simulink model "Battery_model"  (R2021b)
settings: Solver=FixedStepAuto  StartTime=0.0  StopTime=mdl_input.t(end)  FixedStep=1  RelTol=1e-3
values from neighbouring files (symbols this model uses):
  params =     [cell_param.mat]
undefined symbols (not defined in the file or in its folder): mdl_input
libraries: fl_lib x78, nesl_utility x77, simulink x14, ee_lib x14
(part 2 of 2)

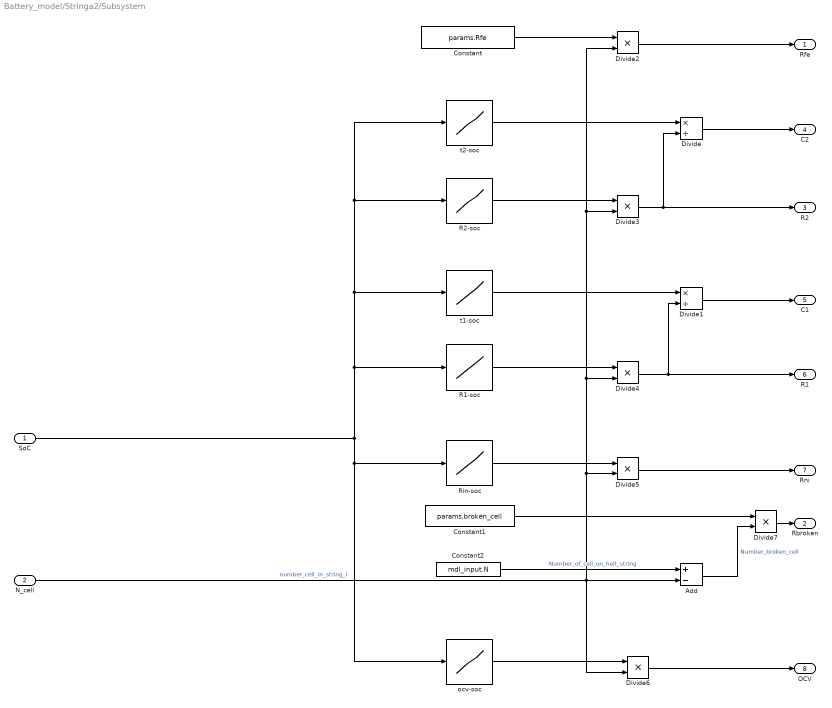
== system Battery_model/Stringa2/Subsystem ==
  SoC : Inport
  N_cell : Inport  Port=2
  Add : Sum  Inputs=+-
  Constant : Constant  Value=params.Rfe
  Constant1 : Constant  Value=params.broken_cell
  Constant2 : Constant  Value=mdl_input.N
  Divide : Product  Inputs=*/
  Divide1 : Product  Inputs=*/
  Divide{2..7} (6 alike) : Product  Inputs=**
  R1-soc : Lookup_n-D  NumberOfTableDimensions=1  BreakpointsForDimension1=params.SoC  Table=params.R1  InternalRulePriority=Speed  RndMeth=Simplest  InputSameDT=on
  R2-soc : Lookup_n-D  NumberOfTableDimensions=1  BreakpointsForDimension1=params.SoC  Table=params.R2  InternalRulePriority=Speed  RndMeth=Simplest  InputSameDT=on
  Rin-soc : Lookup_n-D  NumberOfTableDimensions=1  BreakpointsForDimension1=params.SoC  Table=params.Rni  InternalRulePriority=Speed  RndMeth=Simplest  InputSameDT=on
  ocv-soc : Lookup_n-D  NumberOfTableDimensions=1  BreakpointsForDimension1=params.SoC  Table=params.OCV  ExtrapMethod=Clip  UseLastTableValue=on  InternalRulePriority=Speed  RndMeth=Simplest  InputSameDT=on
  t1-soc : Lookup_n-D  NumberOfTableDimensions=1  BreakpointsForDimension1=params.SoC  Table=params.t1  InternalRulePriority=Speed  RndMeth=Simplest  InputSameDT=on
  t2-soc : Lookup_n-D  NumberOfTableDimensions=1  BreakpointsForDimension1=params.SoC  Table=params.t2  InternalRulePriority=Speed  RndMeth=Simplest  InputSameDT=on
  Rfe : Outport
  Rbroken : Outport  Port=2
  R2 : Outport  Port=3
  C2 : Outport  Port=4
  C1 : Outport  Port=5
  R1 : Outport  Port=6
  Rni : Outport  Port=7
  OCV : Outport  Port=8
  wires:
  SoC/1 -> ocv-soc/1, Rin-soc/1, t1-soc/1, R2-soc/1, t2-soc/1, R1-soc/1
  t1-soc/1 -> Divide1/1
  Divide1/1 -> C1/1
  t2-soc/1 -> Divide/1
  Divide/1 -> C2/1
  Constant/1 -> Divide2/1
  Divide2/1 -> Rfe/1
  R2-soc/1 -> Divide3/1
  Divide3/1 -> Divide/2, R2/1
  Divide4/1 -> Divide1/2, R1/1
  R1-soc/1 -> Divide4/1
  ocv-soc/1 -> Divide6/1
  Divide6/1 -> OCV/1
  Rin-soc/1 -> Divide5/1
  N_cell/1 -> Divide6/2, Add/2, Divide5/2, Divide4/2, Divide3/2, Divide2/2  "number_cell_in_string_i"
  Constant2/1 -> Add/1  "Number_of_cell_on_helt_string"
  Constant1/1 -> Divide7/1
  Add/1 -> Divide7/2  "Number_broken_cell"
  Divide7/1 -> Rbroken/1
  Divide5/1 -> Rni/1

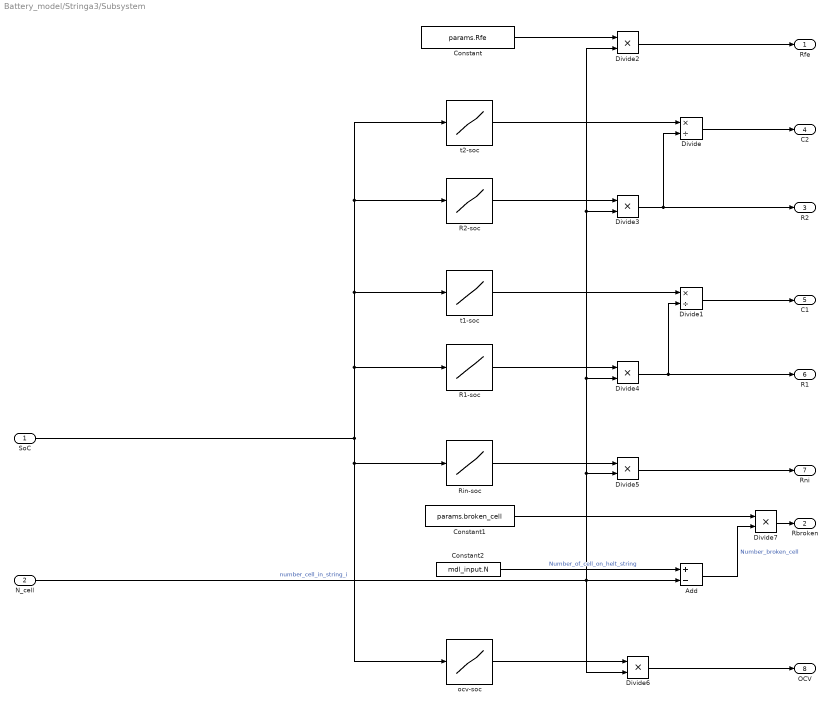
== system Battery_model/Stringa3/Subsystem ==
  SoC : Inport
  N_cell : Inport  Port=2
  Add : Sum  Inputs=+-
  Constant : Constant  Value=params.Rfe
  Constant1 : Constant  Value=params.broken_cell
  Constant2 : Constant  Value=mdl_input.N
  Divide : Product  Inputs=*/
  Divide1 : Product  Inputs=*/
  Divide{2..7} (6 alike) : Product  Inputs=**
  R1-soc : Lookup_n-D  NumberOfTableDimensions=1  BreakpointsForDimension1=params.SoC  Table=params.R1  InternalRulePriority=Speed  RndMeth=Simplest  InputSameDT=on
  R2-soc : Lookup_n-D  NumberOfTableDimensions=1  BreakpointsForDimension1=params.SoC  Table=params.R2  InternalRulePriority=Speed  RndMeth=Simplest  InputSameDT=on
  Rin-soc : Lookup_n-D  NumberOfTableDimensions=1  BreakpointsForDimension1=params.SoC  Table=params.Rni  InternalRulePriority=Speed  RndMeth=Simplest  InputSameDT=on
  ocv-soc : Lookup_n-D  NumberOfTableDimensions=1  BreakpointsForDimension1=params.SoC  Table=params.OCV  ExtrapMethod=Clip  UseLastTableValue=on  InternalRulePriority=Speed  RndMeth=Simplest  InputSameDT=on
  t1-soc : Lookup_n-D  NumberOfTableDimensions=1  BreakpointsForDimension1=params.SoC  Table=params.t1  InternalRulePriority=Speed  RndMeth=Simplest  InputSameDT=on
  t2-soc : Lookup_n-D  NumberOfTableDimensions=1  BreakpointsForDimension1=params.SoC  Table=params.t2  InternalRulePriority=Speed  RndMeth=Simplest  InputSameDT=on
  Rfe : Outport
  Rbroken : Outport  Port=2
  R2 : Outport  Port=3
  C2 : Outport  Port=4
  C1 : Outport  Port=5
  R1 : Outport  Port=6
  Rni : Outport  Port=7
  OCV : Outport  Port=8
  wires:
  SoC/1 -> ocv-soc/1, Rin-soc/1, t1-soc/1, R2-soc/1, t2-soc/1, R1-soc/1
  t1-soc/1 -> Divide1/1
  Divide1/1 -> C1/1
  t2-soc/1 -> Divide/1
  Divide/1 -> C2/1
  Constant/1 -> Divide2/1
  Divide2/1 -> Rfe/1
  R2-soc/1 -> Divide3/1
  Divide3/1 -> Divide/2, R2/1
  Divide4/1 -> Divide1/2, R1/1
  R1-soc/1 -> Divide4/1
  ocv-soc/1 -> Divide6/1
  Divide6/1 -> OCV/1
  Rin-soc/1 -> Divide5/1
  N_cell/1 -> Divide6/2, Add/2, Divide5/2, Divide4/2, Divide3/2, Divide2/2  "number_cell_in_string_i"
  Constant2/1 -> Add/1  "Number_of_cell_on_helt_string"
  Constant1/1 -> Divide7/1
  Add/1 -> Divide7/2  "Number_broken_cell"
  Divide7/1 -> Rbroken/1
  Divide5/1 -> Rni/1

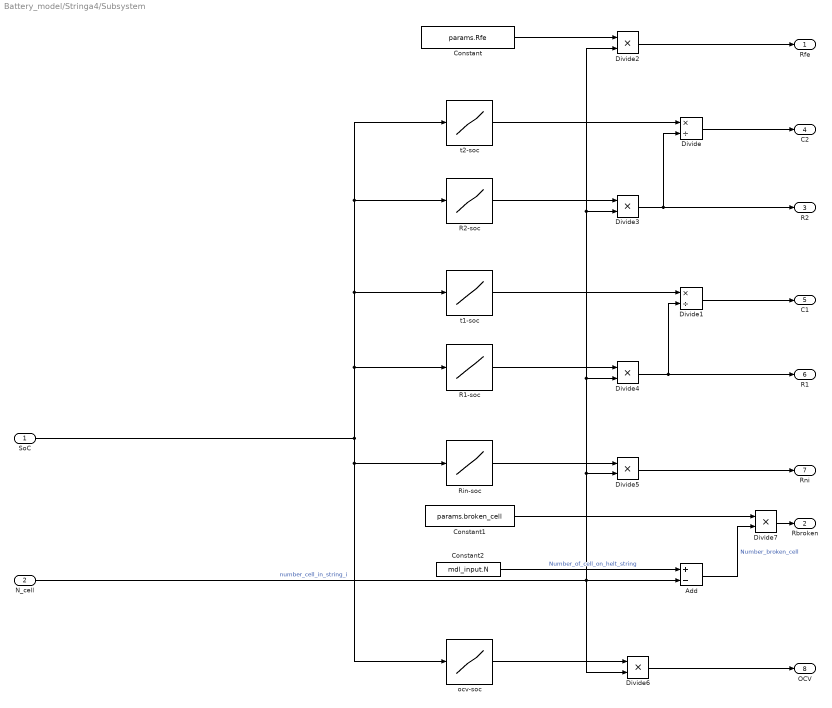
== system Battery_model/Stringa4/Subsystem ==
  SoC : Inport
  N_cell : Inport  Port=2
  Add : Sum  Inputs=+-
  Constant : Constant  Value=params.Rfe
  Constant1 : Constant  Value=params.broken_cell
  Constant2 : Constant  Value=mdl_input.N
  Divide : Product  Inputs=*/
  Divide1 : Product  Inputs=*/
  Divide{2..7} (6 alike) : Product  Inputs=**
  R1-soc : Lookup_n-D  NumberOfTableDimensions=1  BreakpointsForDimension1=params.SoC  Table=params.R1  InternalRulePriority=Speed  RndMeth=Simplest  InputSameDT=on
  R2-soc : Lookup_n-D  NumberOfTableDimensions=1  BreakpointsForDimension1=params.SoC  Table=params.R2  InternalRulePriority=Speed  RndMeth=Simplest  InputSameDT=on
  Rin-soc : Lookup_n-D  NumberOfTableDimensions=1  BreakpointsForDimension1=params.SoC  Table=params.Rni  InternalRulePriority=Speed  RndMeth=Simplest  InputSameDT=on
  ocv-soc : Lookup_n-D  NumberOfTableDimensions=1  BreakpointsForDimension1=params.SoC  Table=params.OCV  ExtrapMethod=Clip  UseLastTableValue=on  InternalRulePriority=Speed  RndMeth=Simplest  InputSameDT=on
  t1-soc : Lookup_n-D  NumberOfTableDimensions=1  BreakpointsForDimension1=params.SoC  Table=params.t1  InternalRulePriority=Speed  RndMeth=Simplest  InputSameDT=on
  t2-soc : Lookup_n-D  NumberOfTableDimensions=1  BreakpointsForDimension1=params.SoC  Table=params.t2  InternalRulePriority=Speed  RndMeth=Simplest  InputSameDT=on
  Rfe : Outport
  Rbroken : Outport  Port=2
  R2 : Outport  Port=3
  C2 : Outport  Port=4
  C1 : Outport  Port=5
  R1 : Outport  Port=6
  Rni : Outport  Port=7
  OCV : Outport  Port=8
  wires:
  SoC/1 -> ocv-soc/1, Rin-soc/1, t1-soc/1, R2-soc/1, t2-soc/1, R1-soc/1
  t1-soc/1 -> Divide1/1
  Divide1/1 -> C1/1
  t2-soc/1 -> Divide/1
  Divide/1 -> C2/1
  Constant/1 -> Divide2/1
  Divide2/1 -> Rfe/1
  R2-soc/1 -> Divide3/1
  Divide3/1 -> Divide/2, R2/1
  Divide4/1 -> Divide1/2, R1/1
  R1-soc/1 -> Divide4/1
  ocv-soc/1 -> Divide6/1
  Divide6/1 -> OCV/1
  Rin-soc/1 -> Divide5/1
  N_cell/1 -> Divide6/2, Add/2, Divide5/2, Divide4/2, Divide3/2, Divide2/2  "number_cell_in_string_i"
  Constant2/1 -> Add/1  "Number_of_cell_on_helt_string"
  Constant1/1 -> Divide7/1
  Add/1 -> Divide7/2  "Number_broken_cell"
  Divide7/1 -> Rbroken/1
  Divide5/1 -> Rni/1

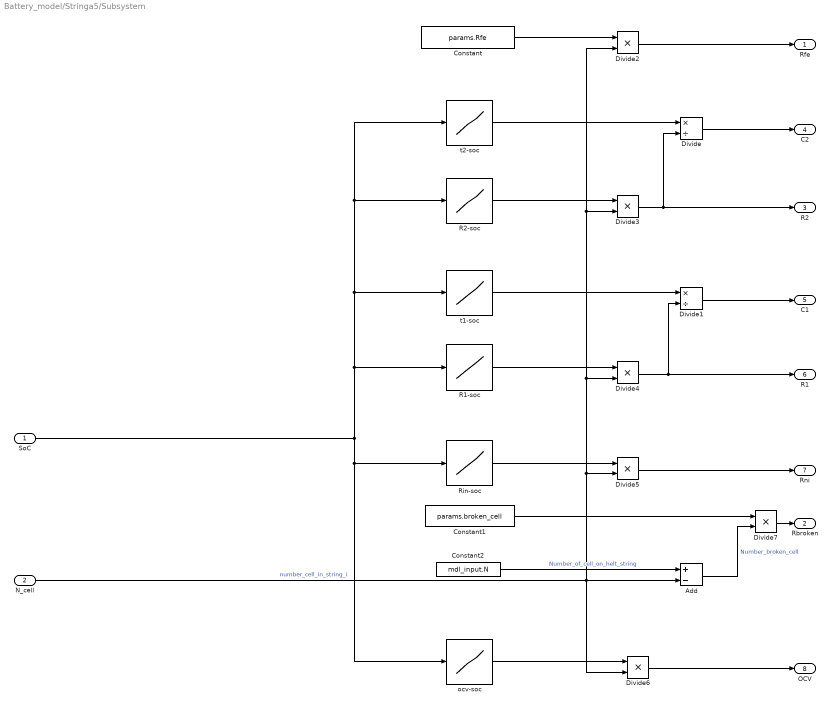
== system Battery_model/Stringa5/Subsystem ==
  SoC : Inport
  N_cell : Inport  Port=2
  Add : Sum  Inputs=+-
  Constant : Constant  Value=params.Rfe
  Constant1 : Constant  Value=params.broken_cell
  Constant2 : Constant  Value=mdl_input.N
  Divide : Product  Inputs=*/
  Divide1 : Product  Inputs=*/
  Divide{2..7} (6 alike) : Product  Inputs=**
  R1-soc : Lookup_n-D  NumberOfTableDimensions=1  BreakpointsForDimension1=params.SoC  Table=params.R1  InternalRulePriority=Speed  RndMeth=Simplest  InputSameDT=on
  R2-soc : Lookup_n-D  NumberOfTableDimensions=1  BreakpointsForDimension1=params.SoC  Table=params.R2  InternalRulePriority=Speed  RndMeth=Simplest  InputSameDT=on
  Rin-soc : Lookup_n-D  NumberOfTableDimensions=1  BreakpointsForDimension1=params.SoC  Table=params.Rni  InternalRulePriority=Speed  RndMeth=Simplest  InputSameDT=on
  ocv-soc : Lookup_n-D  NumberOfTableDimensions=1  BreakpointsForDimension1=params.SoC  Table=params.OCV  ExtrapMethod=Clip  UseLastTableValue=on  InternalRulePriority=Speed  RndMeth=Simplest  InputSameDT=on
  t1-soc : Lookup_n-D  NumberOfTableDimensions=1  BreakpointsForDimension1=params.SoC  Table=params.t1  InternalRulePriority=Speed  RndMeth=Simplest  InputSameDT=on
  t2-soc : Lookup_n-D  NumberOfTableDimensions=1  BreakpointsForDimension1=params.SoC  Table=params.t2  InternalRulePriority=Speed  RndMeth=Simplest  InputSameDT=on
  Rfe : Outport
  Rbroken : Outport  Port=2
  R2 : Outport  Port=3
  C2 : Outport  Port=4
  C1 : Outport  Port=5
  R1 : Outport  Port=6
  Rni : Outport  Port=7
  OCV : Outport  Port=8
  wires:
  SoC/1 -> ocv-soc/1, Rin-soc/1, t1-soc/1, R2-soc/1, t2-soc/1, R1-soc/1
  t1-soc/1 -> Divide1/1
  Divide1/1 -> C1/1
  t2-soc/1 -> Divide/1
  Divide/1 -> C2/1
  Constant/1 -> Divide2/1
  Divide2/1 -> Rfe/1
  R2-soc/1 -> Divide3/1
  Divide3/1 -> Divide/2, R2/1
  Divide4/1 -> Divide1/2, R1/1
  R1-soc/1 -> Divide4/1
  ocv-soc/1 -> Divide6/1
  Divide6/1 -> OCV/1
  Rin-soc/1 -> Divide5/1
  N_cell/1 -> Divide6/2, Add/2, Divide5/2, Divide4/2, Divide3/2, Divide2/2  "number_cell_in_string_i"
  Constant2/1 -> Add/1  "Number_of_cell_on_helt_string"
  Constant1/1 -> Divide7/1
  Add/1 -> Divide7/2  "Number_broken_cell"
  Divide7/1 -> Rbroken/1
  Divide5/1 -> Rni/1
